simulink subsystem "aeroModel"  (R2026a)
settings: Solver=VariableStepAuto
values from neighbouring files (symbols this model uses):
  vehicleParams = 18.0    [plantParams.sldd]
settings Model: DataDictionary=plantParams.sldd  EnableAccessToBaseWorkspace=off  Creator=maxhu  LastModifiedBy=maxhu

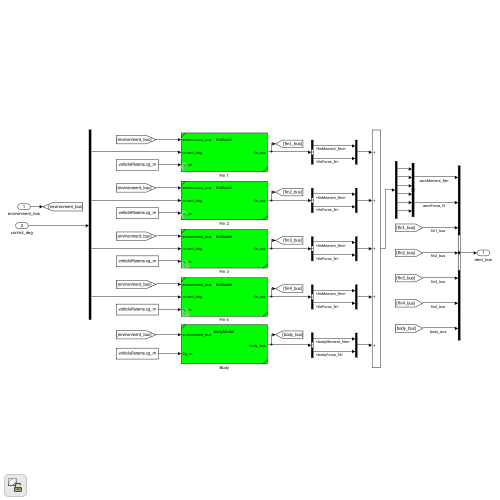
[thumbnail: Simulink's stored preview of the top-level diagram]
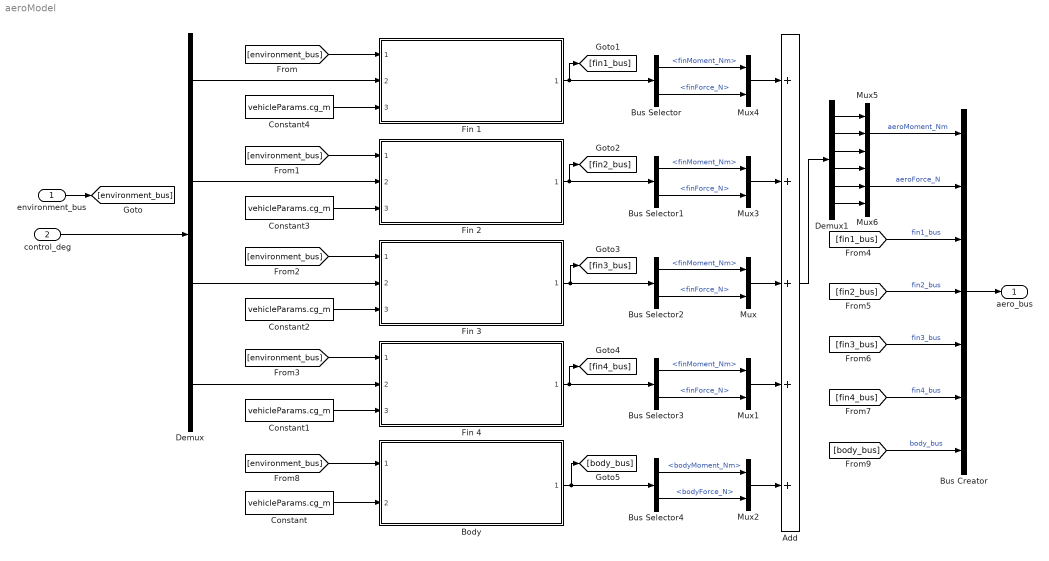
== system aeroModel ==
  environment_bus : Inport
  control_deg : Inport  Port=2
  Add : Sum  Inputs=+++++
  Body : Subsystem  ReferencedSubsystem=bodyModel
      settings: PermitHierarchicalResolution=None
  Bus Creator : BusCreator  Inputs=7
  Bus Selector{,1..3} (4 alike) : BusSelector  OutputSignals=finMoment_Nm,finForce_N
  Bus Selector4 : BusSelector  OutputSignals=bodyMoment_Nm,bodyForce_N
  Constant{,1..4} (5 alike) : Constant  Value=vehicleParams.cg_m
  Demux : Demux
  Demux1 : Demux  Outputs=6
  Fin 1 : Subsystem  ReferencedSubsystem=finModel  finAngles_rad=aeroParams.finAngles1_rad  finCP_m=aeroParams.finCP1_m
      settings: PermitHierarchicalResolution=None
  Fin 2 : Subsystem  ReferencedSubsystem=finModel  finAngles_rad=aeroParams.finAngles2_rad  finCP_m=aeroParams.finCP2_m
      settings: PermitHierarchicalResolution=None
  Fin 3 : Subsystem  ReferencedSubsystem=finModel  finAngles_rad=aeroParams.finAngles3_rad  finCP_m=aeroParams.finCP3_m
      settings: PermitHierarchicalResolution=None
  Fin 4 : Subsystem  ReferencedSubsystem=finModel  finAngles_rad=aeroParams.finAngles4_rad  finCP_m=aeroParams.finCP4_m
      settings: PermitHierarchicalResolution=None
  Mux{,1..4} (5 alike) : Mux  Inputs=2
  Mux5 : Mux  Inputs=3
  Mux6 : Mux  Inputs=3
  aero_bus : Outport
  wires:
  Constant4/1 -> Fin 1/3
  Constant3/1 -> Fin 2/3
  Constant2/1 -> Fin 3/3
  Constant1/1 -> Fin 4/3
  [body_bus] -> Bus Creator/7  "body_bus"
  [fin4_bus] -> Bus Creator/6  "fin4_bus"
  [fin3_bus] -> Bus Creator/5  "fin3_bus"
  [fin2_bus] -> Bus Creator/4  "fin2_bus"
  [fin1_bus] -> Bus Creator/3  "fin1_bus"
  Mux6/1 -> Bus Creator/2  "aeroForce_N"
  Mux5/1 -> Bus Creator/1  "aeroMoment_Nm"
  Demux1/6 -> Mux6/3
  Demux1/5 -> Mux6/2
  Demux1/4 -> Mux6/1
  Demux1/3 -> Mux5/3
  Demux1/2 -> Mux5/2
  Demux1/1 -> Mux5/1
  Add/1 -> Demux1/1
  Mux2/1 -> Add/5
  Mux1/1 -> Add/4
  Mux/1 -> Add/3
  Mux3/1 -> Add/2
  Mux4/1 -> Add/1
  Bus Selector4/2 -> Mux2/2  "<bodyForce_N>"
  Bus Selector4/1 -> Mux2/1  "<bodyMoment_Nm>"
  Fin 4/1 -> [fin4_bus], Bus Selector3/1
  Bus Selector3/2 -> Mux1/2  "<finForce_N>"
  Bus Selector3/1 -> Mux1/1  "<finMoment_Nm>"
  Fin 3/1 -> [fin3_bus], Bus Selector2/1
  Bus Selector2/2 -> Mux/2  "<finForce_N>"
  Bus Selector2/1 -> Mux/1  "<finMoment_Nm>"
  Fin 2/1 -> [fin2_bus], Bus Selector1/1
  Bus Selector1/2 -> Mux3/2  "<finForce_N>"
  Bus Selector1/1 -> Mux3/1  "<finMoment_Nm>"
  Bus Selector/2 -> Mux4/2  "<finForce_N>"
  Bus Selector/1 -> Mux4/1  "<finMoment_Nm>"
  Bus Creator/1 -> aero_bus/1
  Demux/4 -> Fin 4/2
  Demux/3 -> Fin 3/2
  Demux/2 -> Fin 2/2
  Demux/1 -> Fin 1/2
  [environment_bus] -> Fin 4/1
  [environment_bus] -> Fin 3/1
  [environment_bus] -> Fin 2/1
  [environment_bus] -> Fin 1/1
  control_deg/1 -> Demux/1
  environment_bus/1 -> [environment_bus]
  Fin 1/1 -> [fin1_bus], Bus Selector/1
  Body/1 -> Bus Selector4/1, [body_bus]
  [environment_bus] -> Body/1
  Constant/1 -> Body/2
